simulink model "sflib2"  (Simulink 6.2)
settings: Solver=ode45  StartTime=0.0  StopTime=10.0  RelTol=1e-3
settings Model: LastModifiedBy=achimk
settings DebuggingCC: SolverPrmCheckMsg=warning

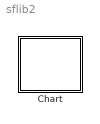
== system sflib2 ==
  Chart : Stateflow chart

== stateflow chart Chart ==
  state SESattention
    \\Sally\LeftCameraAgent\FrameGrabber.ObtainImage()
    \\Sally\SESAgent\ProcessImage()
    \\Sally\SESAgent\CalculateSalience()
    \\Sally\
  state Initial
    \\Sally\LeftCameraAgent\FrameGrabber.Initialize()
    \\Sally\LeftCameraAgent\FrameGrabber.ObtainImage()
    \\Sally\LeftCameraAgent\FrameGrabber.ObtainImage()
  (default) -> Initial : Start
  Initial -> SESattention : Always
  SESattention -> SESattention : Always
